simulink model "Problem6"  (R2020b)
settings: Solver=VariableStepAuto  StartTime=0.0  StopTime=10.0  MaxStep=0.001  RelTol=1e-3
settings Model: OrderedModelArguments=off  Creator=HP  LastModifiedBy=HP

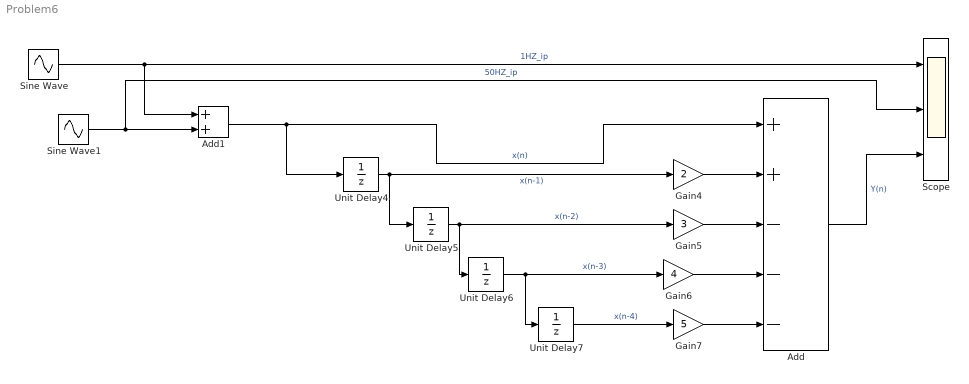
== system Problem6 ==
  Add : Sum  Inputs=++---
  Add1 : Sum
  Gain4 : Gain  Gain=2
  Gain5 : Gain  Gain=3
  Gain6 : Gain  Gain=4
  Gain7 : Gain  Gain=5
  Scope : Scope  NumInputPorts=3
  Sine Wave : Sin  SampleTime=0
  Sine Wave1 : Sin  Frequency=50  SampleTime=0
  Unit Delay{4..7} (4 alike) : UnitDelay  SampleTime=-1  HasFrameUpgradeWarning=on
  wires:
  Sine Wave1/1 -> Scope/2, Add1/2  "50HZ_ip"
  Sine Wave/1 -> Add1/1, Scope/1  "1HZ_ip"
  Unit Delay6/1 -> Gain6/1, Unit Delay7/1  "x(n-3)"
  Add1/1 -> Unit Delay4/1, Add/1  "x(n)"
  Gain7/1 -> Add/5
  Unit Delay5/1 -> Gain5/1, Unit Delay6/1  "x(n-2)"
  Unit Delay7/1 -> Gain7/1  "x(n-4)"
  Gain4/1 -> Add/2
  Gain5/1 -> Add/3
  Gain6/1 -> Add/4
  Add/1 -> Scope/3  "Y(n)"
  Unit Delay4/1 -> Gain4/1, Unit Delay5/1  "x(n-1)"
